simulink model "Spike2018"  (R2018b)
settings: Solver=FixedStepAuto  StartTime=0.0  StopTime=10.0  RelTol=1e-3
undefined symbols (not defined in the file or in its folder): aero, fa, fde, fdelL, fh, fm, idxa, idxde, idxdelL, idxh, idxm
libraries: aerolibconvert2 x4, aerolibasang x3, aerolibadyn x2, shared6dof x1
settings Model: Creator=fberbari  LastModifiedBy=Antho
settings SFSimCC: DefaultCustomCodeFunctionArrayLayout=Row-major
settings RTWCC: GenCodeOnly=on  PackageGeneratedCodeAndArtifacts=on  PackageName=GeneratedCCode.zip  TargetLang=C++
settings GRTTargetCC: TargetLangStandard=C++03 (ISO)  MatFileLogging=off  MultiInstanceERTCode=on  CodeInterfacePackaging=C++ class

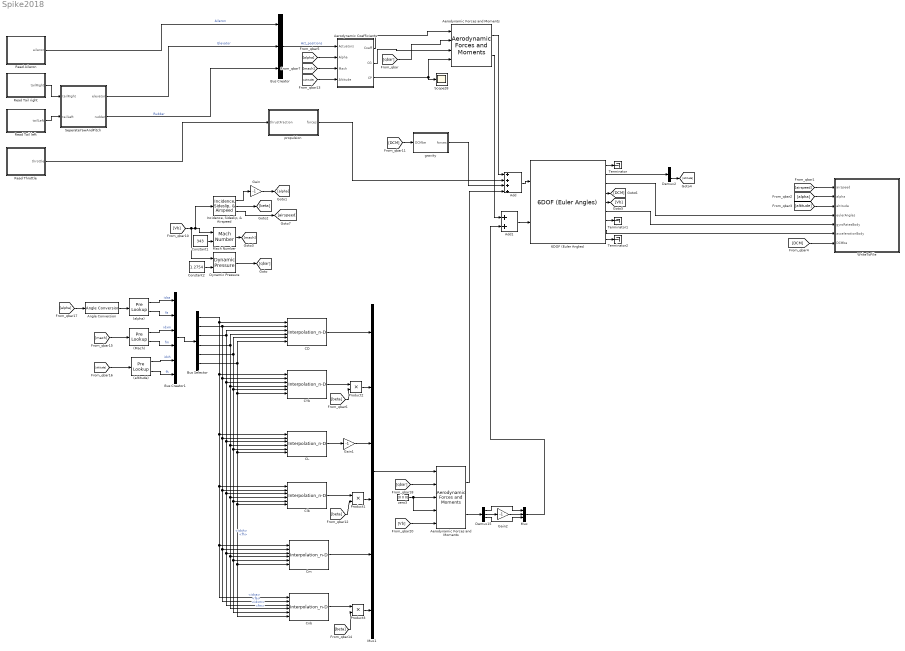
== system Spike2018 ==
  (Mach) : PreLookup  BreakpointsData=aero{1}.mach  BeginIndexSearchUsingPreviousIndexResult=on  ExtrapMethod=Linear  DiagnosticForOutOfRangeInput=Warning  IndexDataTypeStr=int32  FractionDataTypeStr=double
  (alpha) : PreLookup  BreakpointsData=aero{1}.alpha  BeginIndexSearchUsingPreviousIndexResult=on  ExtrapMethod=Linear  DiagnosticForOutOfRangeInput=Warning  IndexDataTypeStr=int32  FractionDataTypeStr=double
  (altitude) : PreLookup  BreakpointsData=aero{1}.alt  BeginIndexSearchUsingPreviousIndexResult=on  ExtrapMethod=Linear  DiagnosticForOutOfRangeInput=Warning  IndexDataTypeStr=int32  FractionDataTypeStr=double
  6DOF (Euler Angles) : shared6dof/6DOF (Euler Angles)  units=Metric (MKS)  mtype=Fixed  rep=Euler Angles  xme_0=[0 0 150]  Vm_0=[20 0 0]  eul_0=[0 0 0]  pm_0=[0 0 0]  mass_0=800  mass_e=0.5  mass_f=2.0  inertia=[1541 0 0; 0 1898 0; 0 0 3199]  inertia_e=eye(3)  inertia_f=2*eye(3)  k_quat=1.0  vre_flag=on  abi_flag=on  aMode=0  xme_statename=''  Vm_statename=''  eul_statename=''  quat_statename=''  pm_statename=''  mass_statename=''
      settings: SourceProductBaseCode=AE
  Add : Sum  Inputs=++++
  Add1 : Sum
  Aerodynamic Coefficients : Subsystem
  Aerodynamic Forces and Moments : aerolibadyn/Aerodynamic Forces and Moments   inputAxes=Wind  outputForceAxes=Body  outputMomentAxes=Body  S=aero{1}.sref  b=aero{1}.blref  cbar=aero{1}.cbar
      settings: SourceProductName=Aerospace Blockset
  "Aerodynamic Forces and Moments " : aerolibadyn/Aerodynamic Forces and Moments   inputAxes=Body  outputForceAxes=Body  outputMomentAxes=Body  S=aero{1}.sref  b=aero{1}.blref  cbar=aero{1}.cbar
      settings: SourceProductName=Aerospace Blockset
  Angle Conversion : aerolibconvert2/Angle Conversion  IU=rad  OU=deg
  Bus Creator : BusCreator  Inputs=3
  Bus Creator1 : BusCreator  Inputs=6
  Bus Selector : BusSelector  OutputSignals=idxa,fa,idxm,fm,idxh,fh
  CD : Interpolation_n-D  NumberOfTableDimensions=3  Table="permute(aero{1}.cd,[1  2  3])"  DiagnosticForOutOfRangeInput=Warning  OutDataTypeStr=double
      settings: InputPortMap=u0,u1,u2,u3,u4,u5
  CL : Interpolation_n-D  NumberOfTableDimensions=3  Table="permute(aero{1}.cl,[1  2  3])"  DiagnosticForOutOfRangeInput=Warning  OutDataTypeStr=double
      settings: InputPortMap=u0,u1,u2,u3,u4,u5
  CYb : Interpolation_n-D  NumberOfTableDimensions=3  Table="permute(aero{1}.cyb,[1  2  3])"  DiagnosticForOutOfRangeInput=Warning  OutDataTypeStr=double
      settings: InputPortMap=u0,u1,u2,u3,u4,u5
  Clb : Interpolation_n-D  NumberOfTableDimensions=3  Table="permute(aero{1}.clb,[1  2  3])"  DiagnosticForOutOfRangeInput=Warning  OutDataTypeStr=double
      settings: InputPortMap=u0,u1,u2,u3,u4,u5
  Cm : Interpolation_n-D  NumberOfTableDimensions=3  Table="permute(aero{1}.cm,[1  2  3])"  DiagnosticForOutOfRangeInput=Warning  OutDataTypeStr=double
      settings: InputPortMap=u0,u1,u2,u3,u4,u5
  Cnb : Interpolation_n-D  NumberOfTableDimensions=3  Table="permute(aero{1}.cnb,[1  2  3])"  DiagnosticForOutOfRangeInput=Warning  OutDataTypeStr=double
      settings: InputPortMap=u0,u1,u2,u3,u4,u5
  Constant1 : Constant  Value=343
  Constant2 : Constant  Value=1.2754
  Demux15 : Demux  Outputs=3
  Demux2 : Demux  Outputs=3
  Dynamic Pressure : aerolibasang/Dynamic Pressure
  Gain : Gain  Gain=-1
  Gain1 : Gain  Gain=-1
  Gain2 : Gain  Gain=-1
  "Incidence, Sideslip, & Airspeed" : aerolibasang/Incidence, Sideslip, & Airspeed
      settings: SourceProductName=Aerospace Blockset
  Mach Number : aerolibasang/Mach Number
      settings: SourceProductName=Aerospace Blockset  SourceProductBaseCode=AE
  Mux : Mux  Inputs=3
  Mux1 : Mux  Inputs=6
  Product1 : Product  RndMeth=Zero
  Product2 : Product  RndMeth=Zero
  Product3 : Product  RndMeth=Zero
  Read Aileron : MATLAB Function  TreatAsAtomicUnit=on
  Read Tail left : MATLAB Function  TreatAsAtomicUnit=on
  Read Tail right : MATLAB Function  TreatAsAtomicUnit=on
  Read Throttle : MATLAB Function  TreatAsAtomicUnit=on
  Scope28 : Scope
  SeperateYawAndPitch : MATLAB Function  TreatAsAtomicUnit=on
  Terminator : Terminator
  Terminator1 : Terminator
  Terminator2 : Terminator
  WriteToFile : MATLAB Function  TreatAsAtomicUnit=on
  gravity : MATLAB Function  TreatAsAtomicUnit=on
  propulsion : MATLAB Function  TreatAsAtomicUnit=on
  zero3 : Constant  Value=[0 0 0]
  wires:
  Read Tail right/1(tailRight) -> SeperateYawAndPitch/1(tailRight)
  Read Tail left/1(tailLeft) -> SeperateYawAndPitch/2(tailLeft)
  Mux/1 -> Add1/2
  Gain2/1 -> Mux/2
  Demux15/1 -> Mux/1
  Demux15/3 -> Mux/3
  Gain1/1 -> Mux1/3
  Demux15/2 -> Gain2/1
  [beta] -> Product1/2
  [Vb] -> Aerodynamic Forces and Moments/5
  Angle Conversion/1 -> (alpha)/1
  "Incidence, Sideslip, & Airspeed"/1 -> Gain/1
  [qbar] -> Aerodynamic Forces and Moments/2
  Bus Selector/6 -> Cnb/6, Cm/6, Clb/6, CL/6, CYb/6, CD/6  "<fh>"
  zero3/1 -> Aerodynamic Forces and Moments/4, Aerodynamic Forces and Moments/3
  Bus Selector/5 -> CD/5, Cnb/5, Cm/5, Clb/5, CL/5, CYb/5  "<idxh>"
  Cm/1 -> Mux1/5
  Product3/1 -> Mux1/6
  Product1/1 -> Mux1/4
  Cnb/1 -> Product3/1
  Product2/1 -> Mux1/2
  Bus Selector/1 -> CD/1, CYb/1, Clb/1, Cnb/1, Cm/1, CL/1  "<idxa>"
  Bus Selector/2 -> CD/2, Cnb/2, Cm/2, Clb/2, CL/2, CYb/2  "<fa>"
  CL/1 -> Gain1/1
  SeperateYawAndPitch/1(elevator) -> Bus Creator/2  "Elevator"
  gravity/1(forces) -> Add/3
  Bus Selector/3 -> CD/3, Cnb/3, Cm/3, Clb/3, CL/3, CYb/3  "<idxm>"
  CD/1 -> Mux1/1
  Bus Selector/4 -> CD/4, Cnb/4, Cm/4, Clb/4, CL/4, CYb/4  "<fm>"
  Read Aileron/1(aileron) -> Bus Creator/1  "Aileron"
  Constant2/1 -> Dynamic Pressure/2
  Add1/1 -> 6DOF (Euler Angles)/2
  [DCM] -> gravity/1(DCMbe)
  6DOF (Euler Angles)/5 -> [Vb]
  Read Throttle/1(throttle) -> propulsion/1(thrustFraction)
  Bus Creator/1 -> Aerodynamic Coefficients/1(Actuators)  "Act_positions"
  Dynamic Pressure/1 -> [qbar]
  "Aerodynamic Forces and Moments "/1 -> Add/1
  6DOF (Euler Angles)/2 -> Demux2/1
  "Incidence, Sideslip, & Airspeed"/2 -> [beta]
  [qbar] -> "Aerodynamic Forces and Moments "/2
  Aerodynamic Coefficients/2(CG) -> "Aerodynamic Forces and Moments "/3
  Add/1 -> 6DOF (Euler Angles)/1
  Mach Number/1 -> [mach]
  [Vb] -> Dynamic Pressure/1, "Incidence, Sideslip, & Airspeed"/1, Mach Number/1
  Clb/1 -> Product1/1
  [beta] -> Product3/2
  Aerodynamic Coefficients/3(CP) -> "Aerodynamic Forces and Moments "/4, Scope28/1
  Aerodynamic Coefficients/1(Coeff) -> "Aerodynamic Forces and Moments "/1
  SeperateYawAndPitch/2(rudder) -> Bus Creator/3  "Rudder"
  Gain/1 -> [alpha]
  [alpha] -> Angle Conversion/1
  (alpha)/1 -> Bus Creator1/1  "idxa"
  Constant1/1 -> Mach Number/2
  (Mach)/1 -> Bus Creator1/3  "idxm"
  Demux2/3 -> [altitude]
  Mux1/1 -> Aerodynamic Forces and Moments/1
  [altitude] -> Aerodynamic Coefficients/4(Altitude)
  [mach] -> Aerodynamic Coefficients/3(Mach)
  [mach] -> (Mach)/1
  (altitude)/1 -> Bus Creator1/5  "idxh"
  CYb/1 -> Product2/1
  Aerodynamic Forces and Moments/2 -> Demux15/1
  "Aerodynamic Forces and Moments "/2 -> Add1/1
  [altitude] -> (altitude)/1
  propulsion/1(forces) -> Add/2
  (altitude)/2 -> Bus Creator1/6  "fh"
  Aerodynamic Forces and Moments/1 -> Add/4
  [alpha] -> Aerodynamic Coefficients/2(Alpha)
  6DOF (Euler Angles)/4 -> [DCM]
  (alpha)/2 -> Bus Creator1/2  "fa"
  [beta] -> Product2/2
  Bus Creator1/1 -> Bus Selector/1
  (Mach)/2 -> Bus Creator1/4  "fm"
  "Incidence, Sideslip, & Airspeed"/3 -> [airspeed]
  [airspeed] -> WriteToFile/1(airspeed)
  [alpha] -> WriteToFile/2(alpha)
  [altitude] -> WriteToFile/3(altitude)
  6DOF (Euler Angles)/8 -> WriteToFile/6(accelerationBody)
  6DOF (Euler Angles)/3 -> WriteToFile/4(eulerAngles)
  6DOF (Euler Angles)/6 -> WriteToFile/5(gyroRatesBody)
  [DCM] -> WriteToFile/7(DCMbe)
  6DOF (Euler Angles)/1 -> Terminator/1
  6DOF (Euler Angles)/7 -> Terminator1/1
  6DOF (Euler Angles)/9 -> Terminator2/1

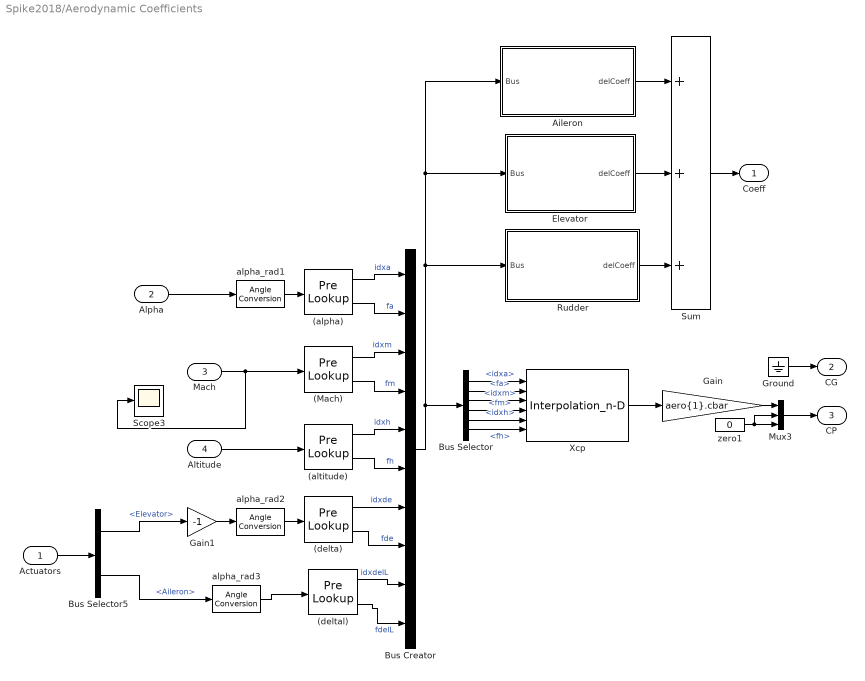
== system Spike2018/Aerodynamic Coefficients ==
  Actuators : Inport
  Alpha : Inport  Port=2
  Mach : Inport  Port=3
  Altitude : Inport  Port=4
  (Mach) : PreLookup  BreakpointsData=aero{1}.mach  BeginIndexSearchUsingPreviousIndexResult=on  ExtrapMethod=Linear  IndexDataTypeStr=int32  FractionDataTypeStr=double
  (alpha) : PreLookup  BreakpointsData=aero{1}.alpha  BeginIndexSearchUsingPreviousIndexResult=on  ExtrapMethod=Linear  IndexDataTypeStr=int32  FractionDataTypeStr=double
  (altitude) : PreLookup  BreakpointsData=aero{1}.alt  BeginIndexSearchUsingPreviousIndexResult=on  ExtrapMethod=Linear  IndexDataTypeStr=int32  FractionDataTypeStr=double
  (delta) : PreLookup  BreakpointsData=aero{1}.delta  BeginIndexSearchUsingPreviousIndexResult=on  ExtrapMethod=Linear  IndexDataTypeStr=int32  FractionDataTypeStr=double
  (deltal) : PreLookup  BreakpointsData=aero{2}.deltal  BeginIndexSearchUsingPreviousIndexResult=on  ExtrapMethod=Linear  IndexDataTypeStr=int32  FractionDataTypeStr=double
  Aileron : Subsystem
  Bus Creator : BusCreator  Inputs=idxa,fa,idxm,fm,idxh,fh,idxde,fde,idxdelL,fdelL
  Bus Selector : BusSelector  OutputSignals=idxa,fa,idxm,fm,idxh,fh
  Bus Selector5 : BusSelector  OutputSignals=Elevator,Aileron
  Elevator : Subsystem
  Gain : Gain  Gain=aero{1}.cbar
  Gain1 : Gain  Gain=-1
  Ground : Ground
  Mux3 : Mux  Inputs=3
  Rudder : Subsystem
  Scope3 : Scope
  Sum : Sum  Inputs=3  SaturateOnIntegerOverflow=on  InputSameDT=on  OutDataTypeStr=Inherit: Same as first input
  Xcp : Interpolation_n-D  NumberOfTableDimensions=3  Table="permute(aero{1}.xcp,[1  2  3])"  OutDataTypeStr=double
      settings: InputPortMap=u0,u1,u2,u3,u4,u5
  alpha_rad1 : aerolibconvert2/Angle Conversion  IU=rad  OU=deg
  alpha_rad2 : aerolibconvert2/Angle Conversion  IU=rad  OU=deg
  alpha_rad3 : aerolibconvert2/Angle Conversion  IU=rad  OU=deg
  zero1 : Constant  Value=0
  Coeff : Outport  InitialOutput=0  VectorParamsAs1DForOutWhenUnconnected=off
  CG : Outport  Port=2  PortDimensions=3  InitialOutput=0  VectorParamsAs1DForOutWhenUnconnected=off
  CP : Outport  Port=3  PortDimensions=3  InitialOutput=0  VectorParamsAs1DForOutWhenUnconnected=off
  wires:
  Sum/1 -> Coeff/1
  Actuators/1 -> Bus Selector5/1
  Ground/1 -> CG/1
  Mux3/1 -> CP/1
  Xcp/1 -> Gain/1
  zero1/1 -> Mux3/2, Mux3/3
  Gain/1 -> Mux3/1
  (alpha)/2 -> Bus Creator/2  "fa"
  (Mach)/2 -> Bus Creator/4  "fm"
  (altitude)/2 -> Bus Creator/6  "fh"
  (altitude)/1 -> Bus Creator/5  "idxh"
  (Mach)/1 -> Bus Creator/3  "idxm"
  (alpha)/1 -> Bus Creator/1  "idxa"
  Bus Selector/1 -> Xcp/1  "<idxa>"
  Bus Selector/2 -> Xcp/2  "<fa>"
  Bus Selector/3 -> Xcp/3  "<idxm>"
  Bus Selector/4 -> Xcp/4  "<fm>"
  Bus Selector/5 -> Xcp/5  "<idxh>"
  Bus Selector/6 -> Xcp/6  "<fh>"
  Bus Creator/1 -> Bus Selector/1, Elevator/1(Bus), Aileron/1(Bus), Rudder/1(Bus)
  Mach/1 -> Scope3/1, (Mach)/1
  Altitude/1 -> (altitude)/1
  alpha_rad1/1 -> (alpha)/1
  Aileron/1(delCoeff) -> Sum/1
  Elevator/1(delCoeff) -> Sum/2
  Rudder/1(delCoeff) -> Sum/3
  (delta)/1 -> Bus Creator/7  "idxde"
  (delta)/2 -> Bus Creator/8  "fde"
  alpha_rad2/1 -> (delta)/1
  Gain1/1 -> alpha_rad2/1
  Bus Selector5/1 -> Gain1/1  "<Elevator>"
  (deltal)/1 -> Bus Creator/9  "idxdelL"
  (deltal)/2 -> Bus Creator/10  "fdelL"
  alpha_rad3/1 -> (deltal)/1
  Bus Selector5/2 -> alpha_rad3/1  "<Aileron>"
  Alpha/1 -> alpha_rad1/1

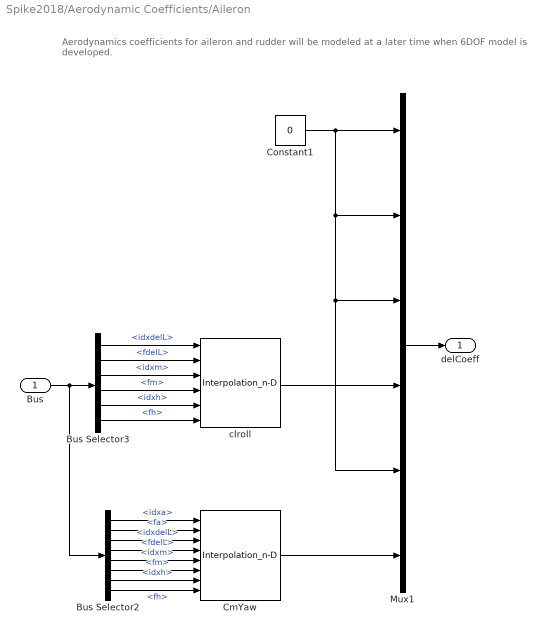
== system Spike2018/Aerodynamic Coefficients/Aileron ==
  note: Aerodynamics coefficients for aileron and rudder will be modeled at a later time when 6DOF model is developed.
  Bus : Inport
  Bus Selector2 : BusSelector  OutputSignals=idxa,fa,idxdelL,fdelL,idxm,fm,idxh,fh
  Bus Selector3 : BusSelector  OutputSignals=idxdelL,fdelL,idxm,fm,idxh,fh
  "CmYaw " : Interpolation_n-D  NumberOfTableDimensions=4  Table=aero{2}.cn_asy  RemoveProtectionIndex=on
      settings: InputPortMap=u0,u1,u2,u3,u4,u5,u6,u7
  Constant1 : Constant  Value=0
  Mux1 : Mux  Inputs=6
  clroll : Interpolation_n-D  NumberOfTableDimensions=3  Table="permute(aero{2}.clroll,[1  2  3])"  RemoveProtectionIndex=on
      settings: InputPortMap=u0,u1,u2,u3,u4,u5
  delCoeff : Outport  VectorParamsAs1DForOutWhenUnconnected=off
  wires:
  Mux1/1 -> delCoeff/1
  Constant1/1 -> Mux1/1, Mux1/2, Mux1/3, Mux1/5
  clroll/1 -> Mux1/4
  Bus/1 -> Bus Selector2/1, Bus Selector3/1
  Bus Selector3/1 -> clroll/1  "<idxdelL>"
  Bus Selector3/2 -> clroll/2  "<fdelL>"
  Bus Selector3/3 -> clroll/3  "<idxm>"
  Bus Selector3/4 -> clroll/4  "<fm>"
  Bus Selector3/5 -> clroll/5  "<idxh>"
  Bus Selector3/6 -> clroll/6  "<fh>"
  "CmYaw "/1 -> Mux1/6
  Bus Selector2/1 -> "CmYaw "/1  "<idxa>"
  Bus Selector2/2 -> "CmYaw "/2  "<fa>"
  Bus Selector2/3 -> "CmYaw "/3  "<idxdelL>"
  Bus Selector2/4 -> "CmYaw "/4  "<fdelL>"
  Bus Selector2/5 -> "CmYaw "/5  "<idxm>"
  Bus Selector2/6 -> "CmYaw "/6  "<fm>"
  Bus Selector2/7 -> "CmYaw "/7  "<idxh>"
  Bus Selector2/8 -> "CmYaw "/8  "<fh>"

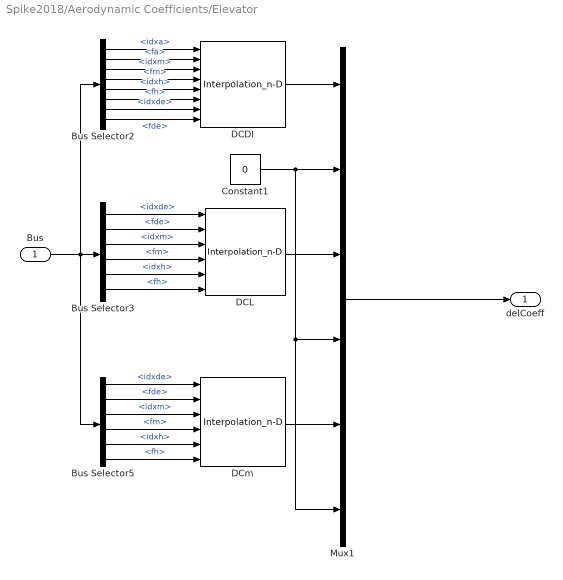
== system Spike2018/Aerodynamic Coefficients/Elevator ==
  Bus : Inport
  Bus Selector2 : BusSelector  OutputSignals=idxa,fa,idxm,fm,idxh,fh,idxde,fde
  Bus Selector3 : BusSelector  OutputSignals=idxde,fde,idxm,fm,idxh,fh
  Bus Selector5 : BusSelector  OutputSignals=idxde,fde,idxm,fm,idxh,fh
  Constant1 : Constant  Value=0
  DCDI : Interpolation_n-D  NumberOfTableDimensions=4  Table=permute(aero{1}.dcdi_sym,[1 3 4 2 ])  RemoveProtectionIndex=on
      settings: InputPortMap=u0,u1,u2,u3,u4,u5,u6,u7
  DCL : Interpolation_n-D  NumberOfTableDimensions=3  Table="permute(aero{1}.dcl_sym,[1  2  3])"  RemoveProtectionIndex=on
      settings: InputPortMap=u0,u1,u2,u3,u4,u5
  DCm : Interpolation_n-D  NumberOfTableDimensions=3  Table="permute(aero{1}.dcm_sym,[1  2  3])"  RemoveProtectionIndex=on
      settings: InputPortMap=u0,u1,u2,u3,u4,u5
  Mux1 : Mux  Inputs=6
  delCoeff : Outport  VectorParamsAs1DForOutWhenUnconnected=off
  wires:
  Mux1/1 -> delCoeff/1
  Bus/1 -> Bus Selector2/1, Bus Selector3/1, Bus Selector5/1
  DCDI/1 -> Mux1/1
  DCL/1 -> Mux1/3
  DCm/1 -> Mux1/5
  Constant1/1 -> Mux1/2, Mux1/4, Mux1/6
  Bus Selector2/1 -> DCDI/1  "<idxa>"
  Bus Selector2/2 -> DCDI/2  "<fa>"
  Bus Selector3/1 -> DCL/1  "<idxde>"
  Bus Selector3/2 -> DCL/2  "<fde>"
  Bus Selector5/1 -> DCm/1  "<idxde>"
  Bus Selector5/2 -> DCm/2  "<fde>"
  Bus Selector2/3 -> DCDI/3  "<idxm>"
  Bus Selector2/4 -> DCDI/4  "<fm>"
  Bus Selector2/5 -> DCDI/5  "<idxh>"
  Bus Selector2/6 -> DCDI/6  "<fh>"
  Bus Selector2/7 -> DCDI/7  "<idxde>"
  Bus Selector2/8 -> DCDI/8  "<fde>"
  Bus Selector3/3 -> DCL/3  "<idxm>"
  Bus Selector3/4 -> DCL/4  "<fm>"
  Bus Selector3/5 -> DCL/5  "<idxh>"
  Bus Selector3/6 -> DCL/6  "<fh>"
  Bus Selector5/3 -> DCm/3  "<idxm>"
  Bus Selector5/4 -> DCm/4  "<fm>"
  Bus Selector5/5 -> DCm/5  "<idxh>"
  Bus Selector5/6 -> DCm/6  "<fh>"

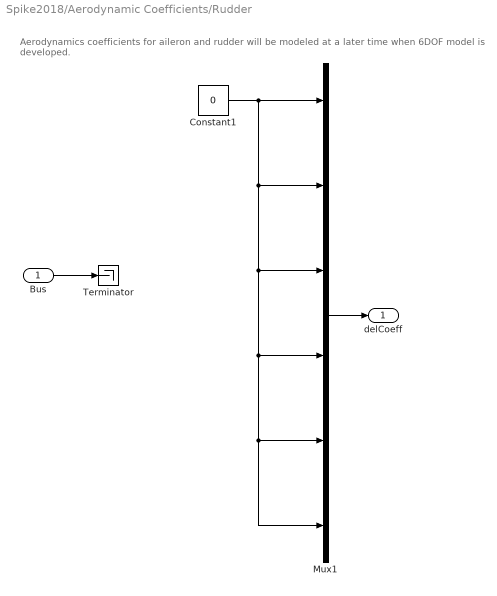
== system Spike2018/Aerodynamic Coefficients/Rudder ==
  note: Aerodynamics coefficients for aileron and rudder will be modeled at a later time when 6DOF model is developed.
  Bus : Inport
  Constant1 : Constant  Value=0
  Mux1 : Mux  Inputs=6
  Terminator : Terminator
  delCoeff : Outport  VectorParamsAs1DForOutWhenUnconnected=off
  wires:
  Mux1/1 -> delCoeff/1
  Constant1/1 -> Mux1/6, Mux1/5, Mux1/4, Mux1/3, Mux1/2, Mux1/1
  Bus/1 -> Terminator/1

== matlab function Spike2018/WriteToFile ==
  data: airspeed input; alpha input; altitude input; eulerAngles input; gyroRatesBody input; accelerationBody input; DCMbe input
%#codegen
function fcn(airspeed, alpha, altitude, eulerAngles, gyroRatesBody, accelerationBody, DCMbe)

mass = 800;
gravityInertial = [0;0;-9.8*mass];
gravityBody = DCMbe * gravityInertial;

airSpeedFile = fopen( 'airspeed.txt', 'a' );

aoaFile = fopen( 'angleOfAttack.txt', 'a' );

altitudeFile = fopen( 'altitude.txt', 'a' );

rollFile = fopen( 'roll.txt', 'a' );
pitchFile = fopen( 'pitch.txt', 'a' );
yawFile = fopen( 'yaw.txt', 'a' );

accXFile = fopen( 'accX.txt', 'a' );
accYFile = fopen( 'accY.txt', 'a' );
accZFile = fopen( 'accZ.txt', 'a' );

gyrXFile = fopen( 'gyrX.txt', 'a' );
gyrYFile = fopen( 'gyrY.txt', 'a' );
gyrZFile = fopen( 'gyrZ.txt', 'a' );

fprintf( airSpeedFile,'%f\n',airspeed);

fprintf( aoaFile,'%f\n',alpha);

fprintf( altitudeFile,'%f\n',altitude);

fprintf( rollFile,'%f\n',eulerAngles(1));
fprintf( pitchFile,'%f\n',eulerAngles(2));
fprintf( yawFile,'%f\n',eulerAngles(3));

fprintf( accXFile,'%f\n',gravityBody(1) + accelerationBody(1));
fprintf( accYFile,'%f\n',gravityBody(2) + accelerationBody(2));
fprintf( accZFile,'%f\n',gravityBody(3) + accelerationBody(3));

fprintf( gyrXFile,'%f\n',gyroRatesBody(1));
fprintf( gyrYFile,'%f\n',gyroRatesBody(2));
fprintf( gyrZFile,'%f\n',gyroRatesBody(3));

fclose('all');

== matlab function Spike2018/Read Aileron ==
  data: aileron output
%#codegen
function aileron = fcn()

A = readfile('aileron.txt');

TF = isstrprop(A, 'wspace');
idx = find(TF);

newestElementIndex = 0;

if size(idx) ~= 0
    newestElementIndex = idx(end - 1); %last whitespace is the last return character
end

newestElementStr = A(newestElementIndex : end);

C = real(str2double(newestElementStr));

fclose('all');

maxAileronDeflect = 0.2618; % radians

aileron = (C * maxAileronDeflect) / 100.0;

== matlab function Spike2018/Read Throttle ==
  data: throttle output
%#codegen
function throttle = fcn()

A = readfile('throttle.txt');

TF = isstrprop(A, 'wspace');
idx = find(TF);

newestElementIndex = 0;

if size(idx) ~= 0
    newestElementIndex = idx(end - 1); %last whitespace is the last return character
end

newestElementStr = A(newestElementIndex : end);

C = real(str2double(newestElementStr));

fclose('all');

throttle = (C / 100.0);

== matlab function Spike2018/Read Tail left ==
  data: tailLeft output
%#codegen
function tailLeft = fcn()

A = readfile('tailLeft.txt');

TF = isstrprop(A, 'wspace');
idx = find(TF);

newestElementIndex = 0;

if size(idx) ~= 0
    newestElementIndex = idx(end - 1); %last whitespace is the last return character
end

newestElementStr = A(newestElementIndex : end);

C = real(str2double(newestElementStr));

fclose('all');

tailLeft = C;

== matlab function Spike2018/Read Tail right ==
  data: tailRight output
%#codegen
function tailRight = fcn()

A = readfile('tailRight.txt');

TF = isstrprop(A, 'wspace');
idx = find(TF);

newestElementIndex = 0;

if size(idx) ~= 0
    newestElementIndex = idx(end - 1); %last whitespace is the last return character
end

newestElementStr = A(newestElementIndex : end);

C = real(str2double(newestElementStr));

fclose('all');

tailRight = C;

== matlab function Spike2018/SeperateYawAndPitch ==
  data: elevator output; rudder output; tailRight input; tailLeft input
%#codegen
function [elevator, rudder]=fcn(tailRight, tailLeft)

tailAngle = pi/4;

elevator = ((tailRight - tailLeft) / (2 * cos(tailAngle)));

rudder = ((tailRight + tailLeft) / (2 * sin(tailAngle)));

maxElevatorDeflect = 0.436; % radians

elevator = (elevator * maxElevatorDeflect) / 100.0;

== matlab function Spike2018/gravity ==
  data: forces output; DCMbe input
%#codegen
function forces  = fcn(DCMbe)

mass = 800;
gravityInertial = [0;0;-9.8*mass];
gravityBody = DCMbe * gravityInertial;

forces = gravityBody;

== matlab function Spike2018/propulsion ==
  data: forces output; thrustFraction input
%#codegen
function forces  = fcn(thrustFraction)

maxThrust = 2200; %Newtons
forces = [maxThrust*thrustFraction;0;0];
